simulink model "solarpanelinvreter"  (R2023b)
settings: Solver=VariableStepAuto  StartTime=0.0  StopTime=30  RelTol=1e-3
libraries: spsSeriesRLCBranchLib x6, spsVoltageMeasurementLib x3, spsDiodeLib x1, spsIGBTDiodeLib x1, spsPVArrayLib x1, spsPWMGenerator2LevelLib x1, spsUniversalBridgeLib x1, spspowerguiLib x1
settings Model: Creator=yashu  LastModifiedBy=yashu

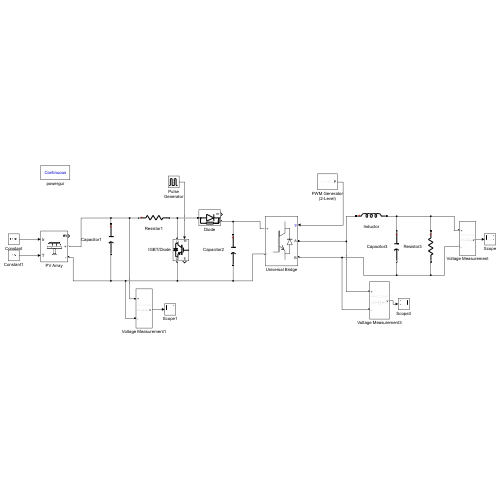
[thumbnail: Simulink's stored preview of the top-level diagram]
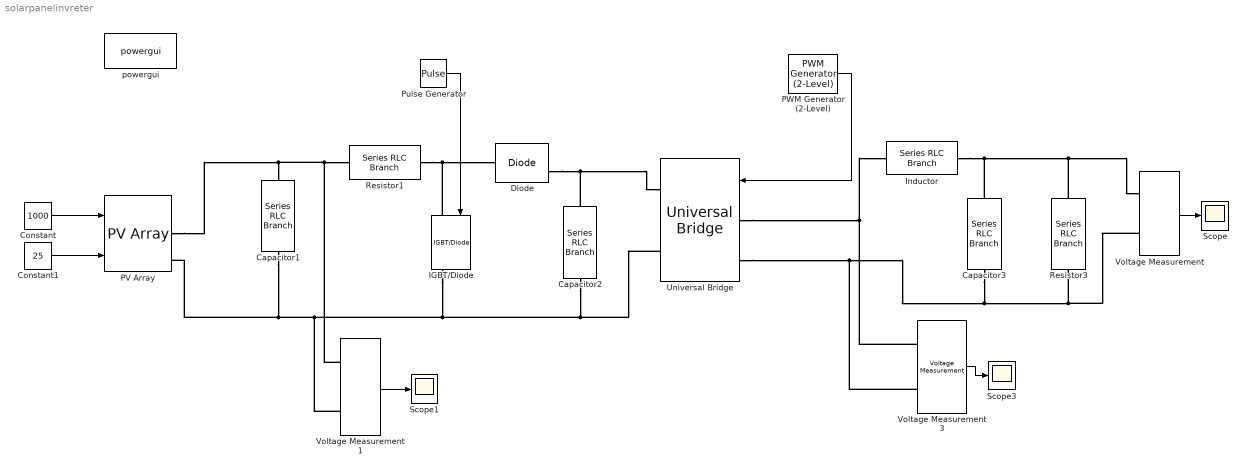
== system solarpanelinvreter ==
  Capacitor1 : spsSeriesRLCBranchLib/Series RLC Branch  LConnTagsString=__new0  RConnTagsString=__new0  BranchType=C  Resistance=1  Inductance=1e-3  SetiL0=off  InitialCurrent=0  Capacitance=0.006  Setx0=off  InitialVoltage=0  Measurements=None
  Capacitor2 : spsSeriesRLCBranchLib/Series RLC Branch  LConnTagsString=__new0  RConnTagsString=__new0  BranchType=C  Resistance=1  Inductance=0.02  SetiL0=off  InitialCurrent=0  Capacitance=0.005  Setx0=off  InitialVoltage=0  Measurements=None
  Capacitor3 : spsSeriesRLCBranchLib/Series RLC Branch  LConnTagsString=__new0  RConnTagsString=__new0  BranchType=C  Resistance=1  Inductance=1e-3  SetiL0=off  InitialCurrent=0  Capacitance=0.0005  Setx0=off  InitialVoltage=0  Measurements=None
  Constant : Constant  Value=1000
  Constant1 : Constant  Value=25
  Diode : spsDiodeLib/Diode  Ron=0.001  Lon=0  Vf=0.8  IC=0  UseSnubber=0  Rs=500  Cs=250e-9  Measurements=on
  IGBT/Diode : spsIGBTDiodeLib/IGBT//Diode  Ron=1e-3  Rs=1e5  Cs=inf  Measurements=on
  Inductor : spsSeriesRLCBranchLib/Series RLC Branch  LConnTagsString=__new0  RConnTagsString=__new0  BranchType=L  Resistance=1  Inductance=0.005  SetiL0=off  InitialCurrent=0  Capacitance=0.005  Setx0=off  InitialVoltage=0  Measurements=None
  PV Array : spsPVArrayLib/PV Array  Npar=20  Nser=5  PlotType=one module @ 25 deg.C & specified irradiances  S_vec=[1000]  Temp_C_vec="[ 25  ]"  ModuleName=Canadian Solar Inc. CS6P-215P  PlotWhenSelected=off  Pm=215.47  Ncell=60  Voc=36.5  Isc=8.01  Vm=29  Im=7.43  beta_Voc_pc=-0.347  alpha_Isc_pc=0.036005  beta_Voc=-0.12665  alpha_Isc=0.002884  IL=8.0291  I0=1.6439e-10  nI=0.96306  Rsh=177.9431  Rs=0.42428  RobustModel=off  RobustCellTemperature=313.3991  BAL=on  Tc=1e-6  Tfilter=5e-5
  PWM Generator (2-Level) : spsPWMGenerator2LevelLib/PWM Generator (2-Level)  ModulatorType=Single-phase full-bridge (4 pulses)  ModulatorMode=Unsynchronized  Fc=27*60  Pc=90  nF=27  MinMax="[ -1  1 ]"  SamplingTechnique=Natural  ModulatingSignals=on  m=0.8  Freq=60  Phase=0  Ts=0  ShowCarrierOutport=off
  Pulse Generator : DiscretePulseGenerator  PulseType=Time based  Period=1/1000  PulseWidth=5
  Resistor1 : spsSeriesRLCBranchLib/Series RLC Branch  LConnTagsString=__new0  RConnTagsString=__new0  BranchType=R  Resistance=1  Inductance=0.02  SetiL0=off  InitialCurrent=0  Capacitance=0.005  Setx0=off  InitialVoltage=0  Measurements=None
  Resistor3 : spsSeriesRLCBranchLib/Series RLC Branch  LConnTagsString=__new0  RConnTagsString=__new0  BranchType=R  Resistance=200  Inductance=1e-3  SetiL0=off  InitialCurrent=0  Capacitance=0.005  Setx0=off  InitialVoltage=0  Measurements=None
  Scope : Scope
  Scope1 : Scope
  Scope3 : Scope
  Universal Bridge : spsUniversalBridgeLib/Universal Bridge  Arms=2  SnubberResistance=1e5  SnubberCapacitance=inf  Device=IGBT / Diodes  Ron=1e-3  Lon=0  ForwardVoltages="[  0  0  ]"  ForwardVoltage=0  GTOparameters=[ 10e-6 , 20e-6 ]  IGBTparameters=[ 1e-6 , 2e-6 ]  Measurements=None  Measurements_2=None  converterType=Rectifier
  Voltage Measurement : spsVoltageMeasurementLib/Voltage Measurement  PhasorSimulation=off  OutputType=Complex  PSBequivalent=0
  Voltage Measurement1 : spsVoltageMeasurementLib/Voltage Measurement  PhasorSimulation=off  OutputType=Complex  PSBequivalent=0
  Voltage Measurement3 : spsVoltageMeasurementLib/Voltage Measurement  PhasorSimulation=off  OutputType=Complex  PSBequivalent=0
  powergui : spspowerguiLib/powergui  Priority=1  SimulationMode=Continuous  SampleTime=50e-6  frequency=60  Iterations=50  frequencyindice=0  Pbase=100e6  ErrMax=1e-4  UnitsV=kV  UnitsW=MW  buscounter=0  FunctionMessages=off  echomessages=off  EnableUseOfTLC=off  CurrentSourceSwitches=off  DisableSnubberDevices=off  DisableRonSwitches=off  DisableVfSwitches=off  DisplayEquations=off  AutomaticDiscreteSolvers=off  SolverType=Tustin/Backward Euler (TBE)  Interpol=off  ExternalGateDelay=off  methode=off  Ts=100  x0status=blocks  SPID=on  SwTol=0  HookPort=off  NonlinearTolerance=1e-4  nMaxIteration=100  ContinueOnMaxIteration=off  RestoreLinks=warning  ResistiveCurrentMeasurement=off  Frange=[0:2:500]  Ylog=off  Xlog=on  ShowGrid=off  save=off  variable=ZData  structure=0  ZoomFFT=off  StartTime=0.0  cycles=1  DisplayStyle=1  fundamental=60  FreqAxis=off  MaxFrequency=1000  frequencyindicesteady=1  RmsSteady=1  display=off
  wires:
  Constant/1 -> PV Array/1
  Constant1/1 -> PV Array/2
  PWM Generator (2-Level)/1 -> Universal Bridge/1
  Voltage Measurement/1 -> Scope/1
  Voltage Measurement1/1 -> Scope1/1
  Voltage Measurement3/1 -> Scope3/1
  Pulse Generator/1 -> IGBT/Diode/1
  connections:
  Voltage Measurement1/LConn1 -- PV Array/RConn1 -- Capacitor1/LConn1 -- Resistor1/LConn1
  Voltage Measurement1/LConn2 -- Universal Bridge/RConn2 -- Capacitor2/RConn1 -- IGBT/Diode/RConn1 -- Capacitor1/RConn1 -- PV Array/RConn2
  Voltage Measurement/LConn2 -- Voltage Measurement3/LConn2 -- Universal Bridge/LConn2 -- Capacitor3/RConn1 -- Resistor3/RConn1
  Resistor3/LConn1 -- Capacitor3/LConn1 -- Inductor/RConn1 -- Voltage Measurement/LConn1
  Universal Bridge/LConn1 -- Inductor/LConn1 -- Voltage Measurement3/LConn1
  Diode/RConn1 -- Capacitor2/LConn1 -- Universal Bridge/RConn1
  Resistor1/RConn1 -- Diode/LConn1 -- IGBT/Diode/LConn1
